simulink model "RLV_Underactuated_BackStepPlusPFL_worksbutidkwhy"  (R2024b)
settings: Solver=FixedStepAuto  StartTime=0.0  StopTime=50  FixedStep=0.0001  RelTol=1e-3
settings Model: Creator=olive  LastModifiedBy=olivermcnaughton
settings DebuggingCC: UnderSpecifiedDimensionMsg=warning

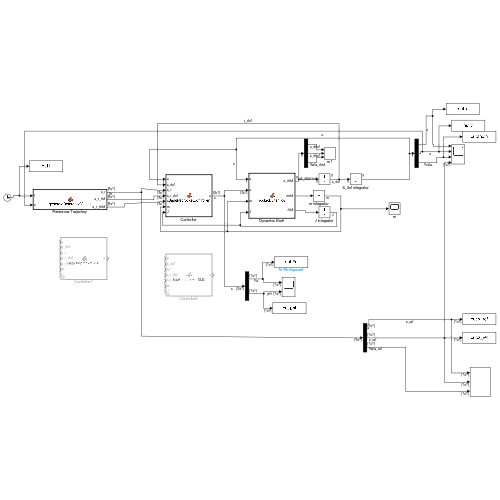
[thumbnail: Simulink's stored preview of the top-level diagram]
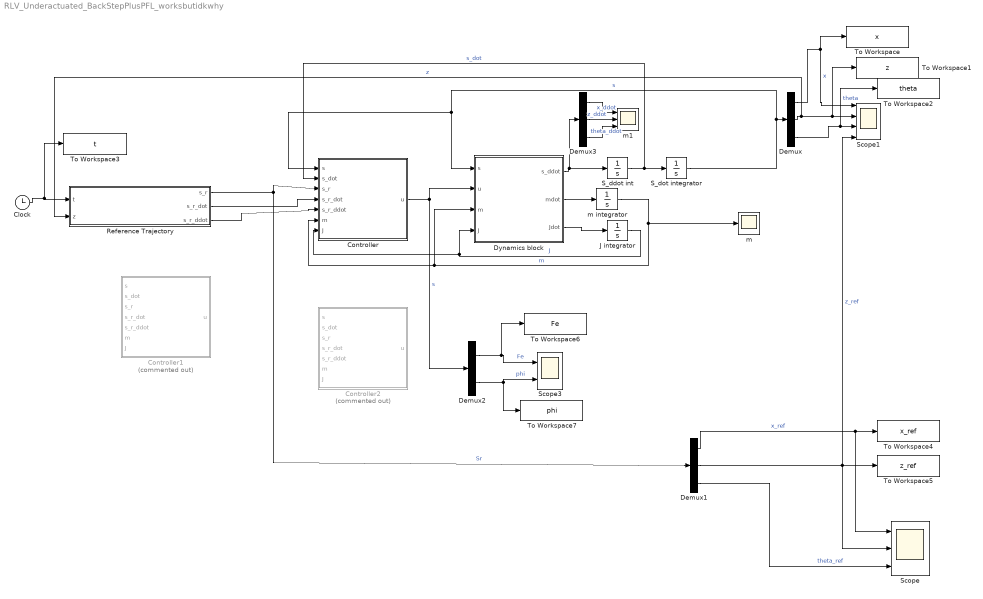
== system RLV_Underactuated_BackStepPlusPFL_worksbutidkwhy ==
  Clock : Clock
  Controller : MATLAB Function  TreatAsAtomicUnit=on
  Controller1 : MATLAB Function  Commented=on  TreatAsAtomicUnit=on
  Controller2 : MATLAB Function  Commented=on  TreatAsAtomicUnit=on
  Demux : Demux  Outputs=3
  Demux1 : Demux  Outputs=3
  Demux2 : Demux  Outputs=2
  Demux3 : Demux  Outputs=3
  Dynamics block : MATLAB Function  TreatAsAtomicUnit=on
  J integrator : Integrator  InitialCondition=5
  Reference Trajectory : MATLAB Function  TreatAsAtomicUnit=on
  S_ddot int : Integrator  InitialCondition=[0; 0; 0]
  S_dot integrator : Integrator  InitialCondition=[0.3;1;0]
  Scope : Scope  NumInputPorts=3
  Scope1 : Scope  NumInputPorts=4
  Scope3 : Scope  NumInputPorts=2
  To Workspace : ToWorkspace  VariableName=x  SaveFormat=Timeseries  SampleTime=-1
  To Workspace1 : ToWorkspace  VariableName=z  SaveFormat=Timeseries  SampleTime=-1
  To Workspace2 : ToWorkspace  VariableName=theta  SaveFormat=Timeseries  SampleTime=-1
  To Workspace3 : ToWorkspace  VariableName=t  SaveFormat=Timeseries  SampleTime=-1
  To Workspace4 : ToWorkspace  VariableName=x_ref  SaveFormat=Timeseries  SampleTime=-1
  To Workspace5 : ToWorkspace  VariableName=z_ref  SaveFormat=Timeseries  SampleTime=-1
  To Workspace6 : ToWorkspace  VariableName=Fe  SaveFormat=Timeseries  SampleTime=-1
  To Workspace7 : ToWorkspace  VariableName=phi  SaveFormat=Timeseries  SampleTime=-1
  m : Scope
  m integrator : Integrator  InitialCondition=25
  m1 : Scope  NumInputPorts=3
  wires:
  Dynamics block/1(s_ddot) -> Demux3/1, S_ddot int/1
  Dynamics block/2(mdot) -> m integrator/1
  Dynamics block/3(Jdot) -> J integrator/1
  S_ddot int/1 -> Controller/2(s_dot), S_dot integrator/1  "s_dot"
  S_dot integrator/1 -> Controller/1(s), Dynamics block/1(s), Demux/1  "s"
  J integrator/1 -> Dynamics block/4(J), Controller/7(J)  "J"
  m integrator/1 -> Dynamics block/3(m), Controller/6(m), m/1  "m"
  Demux/1 -> To Workspace/1, Scope1/1  "x"
  Demux/2 -> Reference Trajectory/2(z), To Workspace1/1, Scope1/2  "z"
  Demux/3 -> To Workspace2/1, Scope1/3  "theta"
  Demux2/2 -> Scope3/2, To Workspace7/1  "phi"
  Demux2/1 -> To Workspace6/1, Scope3/1  "Fe"
  Controller/1(u) -> Demux2/1, Dynamics block/2(u)  "s"
  Clock/1 -> To Workspace3/1, Reference Trajectory/1(t)
  Reference Trajectory/1(s_r) -> Demux1/1, Controller/3(s_r)  "Sr"
  Demux1/2 -> To Workspace5/1, Scope1/4, Scope/2  "z_ref"
  Demux1/1 -> Scope/1, To Workspace4/1  "x_ref"
  Demux1/3 -> Scope/3  "theta_ref"
  Reference Trajectory/2(s_r_dot) -> Controller/4(s_r_dot)
  Demux3/1 -> m1/1  "x_ddot"
  Demux3/2 -> m1/2  "z_ddot"
  Demux3/3 -> m1/3  "theta_ddot"
  Reference Trajectory/3(s_r_ddot) -> Controller/5(s_r_ddot)

== matlab function RLV_Underactuated_BackStepPlusPFL_worksbutidkwhy/Reference Trajectory ==
  data: s_r output; s_r_dot output; t input; z input; s_r_ddot output
function [s_r, s_r_dot, s_r_ddot] = generateReferenceValues(t,z)
% Generates constant reference position and velocity values for x, z, and theta
% Outputs:
%   sr: Reference position vector [x_ref; z_ref; theta_ref]
%   srdot: Reference velocity vector [x_dot_ref; z_dot_ref; theta_dot_ref]

%set position and time for each segment
%set to 1 for a hover, set 0 otherwise
hover = 1;
%set to 1 for a falcon 9 style boost back burn, set 0 otherwise
falcon_9_traj=0;
%set to 1 if tuning
if hover ==1
    x_ref = 10;
    z_ref = 10;
    theta_ref = 0;

    x_dot_ref = 0;
    z_dot_ref = 0;
    theta_dot_ref = 0;

    x_ddot_ref = 0;
    z_ddot_ref = 0;
    theta_ddot_ref = 0;
end

if falcon_9_traj ==1
    %the rocket follows a trajectory of a half sine wave (middle part) then a
    %semi circle for the top of the boostback portion 
    %then a straight line downwards
    %End time of half sinewave
    T1 = 10;
    %End point of half sine wave
    x1 = 30;
    z1 = 40;
    
    %End time of semi circle 
    T2 = 20;
    %End point of semi circle
    x2 = 15; %gives you the position of the other side of the semi circle
    z2 = 40; %this should equal z1
    
    %Landing time of rocket
    T3 = 50;
    %Landing point of rocket
    x3 = 20; % this should be equal to x2
    z3 = 0;
    
    % Initialize reference values for safety
    x_ref = 0;
    z_ref = 0;
    theta_ref = 0;

    x_dot_ref = 0;
    z_dot_ref = 0;
    theta_dot_ref = 0;

    x_ddot_ref = 0;
    z_ddot_ref = 0;
    theta_ddot_ref = 0;

    %The first half sine wave
    if t<T1
        %reference positions
        x_ref = (-sin((pi/2) + pi*t/T1)+1)*x1/2;
        z_ref = z1*t/T1;
        theta_ref = atan(sin(pi*t/T1));
        
        %Reference Velocities
        x_dot_ref = (-pi/T1)*cos((pi/2) + pi*t/T1)*x1/2;
        z_dot_ref = z1/T1;
        theta_dot_ref = (pi/T1)*cos(pi*t/T1)/(sin(pi*t/T1)^2 + 1);

        %Reference Accelerations
        x_ddot_ref = ((pi/T1)^2)*sin((pi/2) + pi*t/T1)*x1/2;
        z_ddot_ref = 0;
        k = pi/T1;
        theta_ddot_ref = -k^2 * sin(k * t) * (3 - sin(k * t)^2) / (1 + sin(k * t)^2)^2;
    end
    %now doing the semi circle
    if t<T2 && t>=T1
        %calculate radius
        r = (x1-x2)/2; %radius 
        h = (x1+x2)/2; %x position for centre of circle
        dT = T2-T1; %Time between points
        dX = x1-x2;
        thetaMax = pi/4; %max angle at when halfway through the semi circle 
        teff = t -T1; %need to "zero" compared to the RHS of the semi circle
        %reference positions
        x_ref = h + r*cos(pi*teff/dT);
        z_ref = z1 + r*sin(pi*teff/dT);
        theta_ref = thetaMax*sin(2*pi*teff/dT + pi);
        %Reference Velocities
        x_dot_ref = (-pi/dT)*r*sin(pi*teff/dT);
        z_dot_ref = (pi/dT)*r*cos(pi*teff/dT);
        theta_dot_ref = thetaMax*(2*pi/dT)*cos(2*pi*teff/dT + pi);

        %Reference Accelerations
        x_ddot_ref = -(pi^2/dT^2)*r*cos(pi*teff/dT);
        z_ddot_ref = -(pi^2/dT^2)*r*sin(pi*teff/dT);
        theta_ddot_ref = -4*(pi^2/dT^2)*thetaMax*sin(pi*teff/dT + pi);
    end
    %now it is landing
    if t>=T2 
        % Position
        x_ref = x2; % Assuming no horizontal movement during landing
        z_ref = z2-4*(t-T2);
        theta_ref = 0; % No rotation during landing
        
        % Velocity
        x_dot_ref = 0;
        if z<10
            z_dot_ref = 0;
            z_ref = 0;
        else 
            z_dot_ref = -4;
        end
        
        theta_dot_ref = 0;
        
        % Acceleration
        x_ddot_ref = 0;
        z_ddot_ref = 0;
        theta_ddot_ref = 0;
    end
    if t>T3
        x_ref = x2;
        z_ref = 0;
        theta_ref = 0; % No rotation during landing
    end
    
end
% Output reference values
s_r = [x_ref; z_ref; theta_ref];
s_r_dot = [x_dot_ref; z_dot_ref; theta_dot_ref];
s_r_ddot = [x_ddot_ref; z_ddot_ref; theta_ddot_ref];
end

== matlab function RLV_Underactuated_BackStepPlusPFL_worksbutidkwhy/Dynamics block ==
  data: s input size=3; u input; m input; J input; s_ddot output size=3; mdot output size=1; Jdot output size=1
function [s_ddot,mdot,Jdot] = rocketDynamics(s,u,m,J)

%initialise states
L1 = 1;
alpha1 = 0.009;
alpha2 = 0.005;
beta = 0.03;
g = 9.81;

%extract states
Fe = u(1);
phi = u(2);

theta = s(3);

%find mdot and Jdot
mdot = -alpha1*(beta*Fe);
Jdot = -alpha2*(beta*Fe);
%update mdot and Jdot

x_ddot = Fe*sin(theta + phi)/m;
z_ddot = -g + Fe*cos(theta+phi)/m; 
theta_ddot = Fe*sin(phi)*(L1)/J;

s_ddot = [x_ddot;z_ddot;theta_ddot];

end

== matlab function RLV_Underactuated_BackStepPlusPFL_worksbutidkwhy/Controller1 ==
  data: s input; s_dot input; s_r input; s_r_dot input; s_r_ddot input; m input; J input; u output
function u = BacksteprocketSMC(s, s_dot, s_r, s_r_dot, s_r_ddot, m, J)
% rocketController - Backstepping-based controller with Sliding Mode Control (SMC)
%
% Inputs:
%   s     - Current state vector [x; z; theta; x_dot; z_dot; theta_dot]
%   s_r   - Reference state vector [x_ref; z_ref; theta_ref]
%   s_r_dot  - Reference velocity vector [x_dot_ref; z_dot_ref; theta_dot_ref]
%   s_r_ddot - Reference acceleration vector [x_ddot_ref; z_ddot_ref; theta_ddot_ref]
%   m     - Current mass of the rocket
%   J     - Current moment of inertia
%
% Output:
%   u     - Control input vector [Fe; phi]

% Constants
g = 9.81; % Gravity

% Extract current states
x = s(1); z = s(2); theta = s(3);
x_dot = s_dot(1); z_dot = s_dot(2); theta_dot = s_dot(3);

% Extract reference states
x_ref = s_r(1); z_ref = s_r(2); theta_ref = s_r(3);
x_dot_ref = s_r_dot(1); z_dot_ref = s_r_dot(2); theta_dot_ref = s_r_dot(3);
x_ddot_ref = s_r_ddot(1); z_ddot_ref = s_r_ddot(2); theta_ddot_ref = s_r_ddot(3);

% Control gains (Backstepping)
kpx = 1; kdx = 1;
kpz = 1; kdz = 1;
kpt = 1; kdt = 1;

% Sliding mode control gains
ksx = 2; 
ksz = 2; 
kst = 2;  % Sliding surface gains
eta_x = 5; 
eta_z = 5; 
eta_theta = 5;  % Control effort gains

% Compute errors
ex = x - x_ref; ez = z - z_ref; et = theta - theta_ref;
edotx = x_dot - x_dot_ref; edotz = z_dot - z_dot_ref; edot_t = theta_dot - theta_dot_ref;

% Define sliding surfaces
s_x = edotx + ksx * ex; %sliding surface for x
s_z = edotz + ksz * ez; %sliding surface for z
s_theta = edot_t + kst * et; %sliding surface for theta

% Equivalent Control (Backstepping)
ax_eq = x_ddot_ref - kpx * ex - kdx * edotx - kpt * et - kdt * edot_t;
az_eq = z_ddot_ref - kpz * ez - kdz * edotz - kpt * et - kdt * edot_t;

% Sliding Mode Switching Control
sat_x = tanh(s_x / 0.1); % Sigmoid approximation of sign function to reduce chattering
sat_z = tanh(s_z / 0.1);
sat_theta = tanh(s_theta / 0.1);

ax_smc = -eta_x * sat_x;
az_smc = -eta_z * sat_z;
theta_smc = -eta_theta * sat_theta; % Additional torque correction

% Total acceleration command (Backstepping + SMC)
ax = ax_eq + ax_smc;
az = az_eq + az_smc;

% Avoid division by zero
denominator = az + g;
if abs(denominator) < 1e-7
    denominator = sign(denominator) * 1e-7;
end

% Compute thrust angle and force
phi = atan2(ax, denominator) - theta + theta_smc; % SMC correction added
Fe = m * sqrt(ax^2 + (az + g)^2); % Ensuring proper force calculation

% Output control vector
u = [Fe; phi];

end

== matlab function RLV_Underactuated_BackStepPlusPFL_worksbutidkwhy/Controller ==
  data: s input; s_dot input; s_r input; s_r_dot input; s_r_ddot input; m input; J input; u output
function u = BacksteprocketController(s, s_dot, s_r, s_r_dot, s_r_ddot, m, J)
% Not sure exactly why this works but it does 
% rocketController - Backstepping-based controller for rocket dynamics
%
% Inputs:
%   s     - Current state vector [x; z; theta; x_dot; z_dot; theta_dot]
%   s_ref - Reference state vector [x_ref; z_ref; x_dot_ref; z_dot_ref; x_ddot_ref; z_ddot_ref]
%   m     - Current mass of the rocket
%   J     - Current moment of inertia
%   gains - Struct containing control gains (k1, k2, k3, k4)
%
% Output:
%   u     - Control input vector [Fe; phi]

% Define bounds
FE_min = 0;   % Lower bound for FE
FE_max = 500; % Upper bound for FE

phi_min = -pi/6;  % Lower bound for phi
phi_max = pi/6;   % Upper bound for phi

%Constants
g = 9.81; % Gravity

% Extract current states
x = s(1);
z = s(2);
theta = s(3);
x_dot = s_dot(1);
z_dot = s_dot(2);
theta_dot = s_dot(3);

% Extract reference states
x_ref = s_r(1);
z_ref = s_r(2);
theta_ref = s_r(3);

x_dot_ref = s_r_dot(1);
z_dot_ref = s_r_dot(2);
theta_dot_ref = s_r_dot(3);

x_ddot_ref = s_r_ddot(1);
z_ddot_ref = s_r_ddot(2);
theta_ddot_ref = s_r_ddot(3);

% Control gains
kpx = 2;
kdx = 5;
kpz = 2;
kdz = 5;

kpt = 1;
kdt = 1;

% Step 1: Compute errors
ex = x - x_ref;
ez = z - z_ref;
et = theta - theta_ref;

edotx = x_dot - x_dot_ref;
edotz = z_dot - z_dot_ref;
edot_t = theta_dot - theta_dot_ref;

% Desired acceleration 
ax = x_ddot_ref - kpx * ex - kdx * edotx;
az = z_ddot_ref - kpz * ez - kdz * edotz;

%check if divide by zero error present
denominator = az+g;

% Avoid division by zero
if abs(denominator) < 1e-6
    denominator = sign(denominator) * 1e-6;
end

phi_cmd = atan2(ax,denominator) - theta;
Fe = m*sqrt(ax^2 + (az+g)^2); % direction of control signal lost 
phi = phi_cmd  - kpt*et - kdt*edot_t; %2nd loop controlling orientation

%bound them within physical limits
Fe = max(FE_min, min(Fe, FE_max));
phi = max(phi_min, min(phi, phi_max));
% Output control vector
u = [Fe; phi];

end

== matlab function RLV_Underactuated_BackStepPlusPFL_worksbutidkwhy/Controller2 ==
  data: s input; s_dot input; s_r input; s_r_dot input; s_r_ddot input; m input; J input; u output
function u = BacksteprocketSMC(s, s_dot, s_r, s_r_dot, s_r_ddot, m, J)
% BacksteprocketSMC - Example of a backstepping + SMC-based controller
% for a rocket with thrust vectoring in 2D.
%
% Inputs:
%   s         - Current state vector [x; z; theta]
%   s_dot     - Current velocities [x_dot; z_dot; theta_dot]
%   s_r       - Reference states [x_ref; z_ref; theta_ref]  (theta_ref may be ignored here)
%   s_r_dot   - Reference velocities [x_dot_ref; z_dot_ref; theta_dot_ref]
%   s_r_ddot  - Reference accelerations [x_ddot_ref; z_ddot_ref; theta_ddot_ref]
%   m         - Rocket mass
%   J         - Rocket moment of inertia
%
% Outputs:
%   u         - Control input [F_e; phi] where
%               F_e  = commanded thrust magnitude
%               phi  = nozzle deflection relative to rocket body
%
% NOTE: This example assumes:
%   1) Thrust direction = (theta + phi).
%   2) Torque tau ~ F_e * L * phi for small phi (L is a pivot arm).
%   3) We do SMC on translational states to get desired net accel (=> alpha, F_e).
%   4) We do SMC on attitude to track alpha. 
%
%   You will need to adapt or refine this to match your actual rocket geometry.

    % Gravity
    g = 9.81;

    % Extract current states
    x       = s(1);
    z       = s(2);
    theta   = s(3);

    x_dot       = s_dot(1);
    z_dot       = s_dot(2);
    theta_dot   = s_dot(3);

    % Extract references (though we won't fully use theta_ref in this example)
    x_ref       = s_r(1);
    z_ref       = s_r(2);
    % theta_ref = s_r(3);  % (Optional if you want separate attitude tracking)

    x_dot_ref   = s_r_dot(1);
    z_dot_ref   = s_r_dot(2);

    x_ddot_ref  = s_r_ddot(1);
    z_ddot_ref  = s_r_ddot(2);
    % theta_ddot_ref = s_r_ddot(3);

    %-------------------------------
    % 1) TRANSLATIONAL SMC
    %-------------------------------
    % Gains for x,z sliding surfaces
    kx   = 2;   % slope in s_x
    kz   = 2;   % slope in s_z
    etaX = 5;   % switching gain for x
    etaZ = 5;   % switching gain for z

    % Errors for x and z
    ex    = x - x_ref;
    ez    = z - z_ref;
    edotx = x_dot - x_dot_ref;
    edotz = z_dot - z_dot_ref;

    % Define sliding surfaces
    s_x = edotx + kx*ex; 
    s_z = edotz + kz*ez;

    % "Equivalent" control for each axis 
    % We want s_x_dot ~ 0 => \ddot{x} = x_ddot_ref - kx \dot{e}_x, ignoring switching
    a_x_eq = x_ddot_ref - kx * edotx;

    % Similarly for z: \ddot{z} + k_z \dot{e}_z = z_ddot_ref
    a_z_eq = z_ddot_ref - kz * edotz;

    % Sliding-mode switching terms
    % Using tanh(...) as a smoothed sign function
    sat_x     = tanh(s_x / 0.1);
    sat_z     = tanh(s_z / 0.1);
    a_x_smc   = -etaX * sat_x;
    a_z_smc   = -etaZ * sat_z;

    % Total commanded accelerations in inertial frame
    a_x_cmd = a_x_eq + a_x_smc;
    a_z_cmd = a_z_eq + a_z_smc;

    %-------------------------------
    % 2) COMPUTE DESIRED THRUST
    %-------------------------------
    % Net vertical + gravity => a_z_cmd + g
    % Magnitude of thrust needed:
    F_e = m * sqrt( a_x_cmd^2 + (a_z_cmd + g)^2 );
    
    % If it is extremely small, avoid division by zero
    if F_e < 1e-6
        F_e = 1e-6;
    end

    %-------------------------------
    % 3) DESIRED THRUST ANGLE
    %-------------------------------
    % The net thrust direction from the vertical is:
    alpha_des = atan2(a_x_cmd, a_z_cmd + g);
    % i.e. if alpha_des>0, thrust is "tilted" to push in +x direction.

    %-------------------------------
    % 4) ATTITUDE SMC
    %-------------------------------
    % We want the rocket's pitch theta to track alpha_des.
    % Define attitude error (rocket pitch minus desired tilt)
    e_theta     = theta - alpha_des;       % current minus desired
    e_theta_dot = theta_dot - 0;           % we want to hold zero relative rate

    % Sliding surface for attitude
    kt = 2;              % slope for s_theta
    s_theta = e_theta_dot + kt * e_theta;

    % Gains for attitude SMC
    eta_theta = 5;       % switching gain for attitude

    % "Equivalent" torque portion: we want \dot{s}_theta = 0 => J*theta_ddot ...
    % For brevity: set eq. part = -kt * e_theta_dot (or use more advanced design)
    alpha_eq  = -kt * e_theta_dot;

    % SMC switching term
    sat_theta = tanh(s_theta / 0.1);
    alpha_smc = -eta_theta * sat_theta;    % additional angular accel

    % Net desired angular acceleration
    theta_ddot_cmd = alpha_eq + alpha_smc;

    % So the torque is:
    tau = J * theta_ddot_cmd;

    %--------------------------------
    % 5) RELATE TORQUE TO NOZZLE ANGLE PHI
    %--------------------------------
    % Suppose torque = F_e * L * sin(phi).
    % For small phi, tau ~ F_e * L * phi, so
    %
    %     phi ~ tau / (F_e * L)
    %
    % If we do not know the pivot arm L, assume L=1 for demonstration:
    L = 1.0;

    % Compute the small nozzle deflection needed to create torque tau
    phi_smc = tau / (F_e * L);

    % The *basic* nozzle angle to produce alpha_des is (alpha_des - theta).
    % Because net thrust direction = theta + phi.
    % Then we add the small correction phi_smc to handle SMC torque. 
    % In many derivations, you would unify these. For a small-angle pivot,
    % you can do a simple sum:
    phi_basic = alpha_des - theta;

    % Combine the two.  You may need to be careful not to double-count
    % angles if your geometry is more complicated:
    phi = phi_basic + phi_smc;

    % Optionally limit phi to some range, e.g. +/- 30 degrees
    maxAngle = 30 * pi/180;
    if abs(phi) > maxAngle
        phi = sign(phi)*maxAngle;
    end

    %-------------------------------
    % 6) Final output
    %-------------------------------
    u = [F_e; phi];
end
